simulink model "EMPlanner_cs"  (R2020a)
settings: Solver=ode5  StartTime=0.0  StopTime=30  FixedStep=1/1000  RelTol=1e-3
PreLoadFcn:
  | mbxruntime.callbacks.PreLoadFcn(bdroot);
PostLoadFcn:
  | mbxruntime.callbacks.PostLoadFcn(bdroot);
InitFcn:
  | mbxruntime.callbacks.InitFcn(bdroot);
StartFcn:
  | mbxruntime.callbacks.StartFcn(bdroot);
StopFcn:
  | mbxruntime.callbacks.StopFcn(bdroot);
model workspace (MAT data in the model file):
  mbox_table : object (value not decoded)
  model_closed = 0
  sim_status = 0
values from neighbouring files (symbols this model uses):
  aubr = [-8 -7.95 -7.9 -7.85 -7.8 -7.75 -7.7 -7.65 -7.6 -7.55 -7.5 -7.45 ... (261 elements, 1x261)]    [table_calibration.mat]
  tablebr = [-1.5 -1.5 -6.69193204056 -6.72439369683 -6.74529114616 -6.75462438856 -6.75239342402 -6.74076432593 -6.71187451024 -6.7106900587 -6.78609036519 -6.73359919607 ... (261261 elements, 1001x261)]    [table_calibration.mat]
  vubr = [0 0.05 0.1 0.15 0.2 0.25 0.3 0.35 0.4 0.45 0.5 0.55 ... (1001 elements, 1x1001)]    [table_calibration.mat]
undefined symbols (not defined in the file or in its folder): c_factor, cf, cr, DiscIntNeverNeededParam, global_path_x, global_path_y, KD_PID_distance, KD_PID_speed, KI_PID_distance, KI_PID_speed, KP_PID_distance, KP_PID_speed, la, lb, LQR_K1, LQR_K2, LQR_K3, LQR_K4, m, rack_displacement, right_wheel_ground, vx_break_point, warningInitialVelocity, x0
libraries: PreScanSimulinkLibrary x39, simulink x19, simulink_extras x11, Solver_SF x1
(part 1 of 11)
CloseFcn:
  | mbxruntime.callbacks.CloseFcn(bdroot);
settings Model: EnablePacing=on  PacingRate=1000  Creator=PRESCAN  LastModifiedBy=vincentwong
settings DataIOCC: LimitDataPoints=on  SaveFormat=Array  ReturnWorkspaceOutputs=off
settings OptimizationCC: ExpressionDepthLimit=2147483647  InitFltsAndDblsToZero=on  LifeSpan=inf
settings DebuggingCC: SaveWithParameterizedLinksMsg=none  UnderspecifiedInitializationDetection=Classic  MergeDetectMultiDrivingBlocksExec=none  SignalResolutionControl=TryResolveAllWithWarning  MultiTaskDSMMsg=warning  MultiTaskCondExecSysMsg=none  FcnCallInpInsideContextMsg=warning  StateNameClashWarn=warning  SFUnexpectedBacktrackingDiag=warning  SFNoUnconditionalDefaultTransitionDiag=warning  SFExecutionAtInitializationDiag=none  ArithmeticOperatorsInVariantConditions=warning
settings HardwareCC: ProdBitPerPointer=32  ProdBitPerSizeT=32  ProdBitPerPtrDiffT=32  ProdLargestAtomicFloat=None  ProdIntDivRoundTo=Undefined  ProdEndianess=Unspecified  ProdWordSize=32  ProdHWDeviceType=32-bit Generic
settings ModelReferenceCC: UpdateModelReferenceTargets=IfOutOfDate  PropagateSignalLabelsOutOfModel=off
settings SFSimCC: SimUseLocalCustomCode=off  SimParseCustomCode=off  CustomCodeUndefinedFunction=UseInterfaceOnly
settings SFSimCC: SimCustomHeaderCode=|
  | #include "prescan.h"
  | #include "prescan_platform.h"
settings RTWCC: RTWUseLocalCustomCode=off
settings CodeAppCC: StateflowObjectComments=on
settings GRTTargetCC: TargetFcnLib=ansi_tfl_tmw.mat  TargetLangStandard=C89/C90 (ANSI)  CombineOutputUpdateFcns=off  GRTInterface=on
settings ConfigComp: CovMetricSettings=dw  CovSaveCumulativeToWorkspaceVar=on  CovSaveSingleToWorkspaceVar=on  CovExternalEMLEnable=off

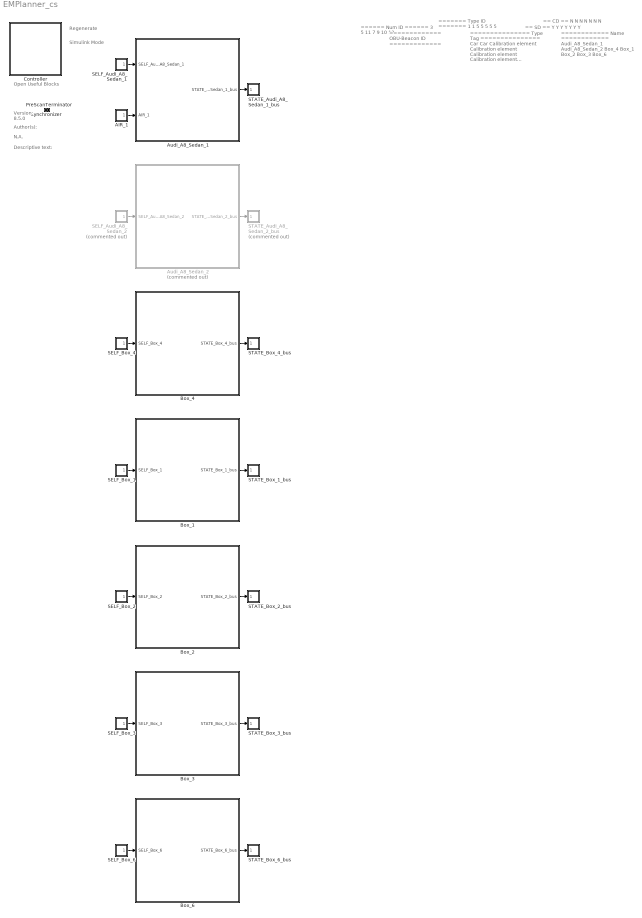
== system EMPlanner_cs ==
  note: Regenerate
  note: Simulink Mode
  note: Open Useful Blocks
  note: 8.5.0
  note: Version:
  note: Author(s):
  note: N.A.
  note: Descriptive text:
  note: ======
      | Num ID
      | ======
      | 3
      | 5
      | 11
      | 7
      | 9
      | 10
      | 13
  note: =============
      | OBU-Beacon ID
      | =============
  note: =======
      | Type ID
      | =======
      | 1
      | 1
      | 5
      | 5
      | 5
      | 5
      | 5
  note: ===============
      | Type Tag
      | ===============
      | Car
      | Car
      | Calibration element
      | Calibration element
      | Calibration element
      | Calibration element
      | Calibration element
  note: ==
      | SD
      | ==
      | Y
      | Y
      | Y
      | Y
      | Y
      | Y
      | Y
  note: ==
      | CD
      | ==
      | N
      | N
      | N
      | N
      | N
      | N
      | N
  note: ============
      | Name
      | ============
      | Audi_A8_Sedan_1
      | Audi_A8_Sedan_2
      | Box_4
      | Box_1
      | Box_2
      | Box_3
      | Box_6
  AIR_1 : Subsystem  Tag=sensor/AIR  Priority=3  LoadFcn=load('PrescanAIRSensorData.mat');load('PrescanAIRSensorMessage.mat')  mask(PreScan Source Block: Actor Independent Receiver (AIR)){}
      mask help:
      | The Actor Information Receiver sensor provides a fast, simple and generic detection solution which is not tied up to a specific technology. The AIR detects the intersection point of the bounding box with the straight line from the sensor axis system to the middle of the bounding box.
      |
      | For more information, please click Help.
      settings: OpenFcn=open_system([gcb '/Sensor'],'mask')
      mask Help: eval('openHelp(413)')
      mask Display: image(imread('AIR.png'))
  Audi_A8_Sedan_1 : Subsystem  Tag=WorldObjectSubSystem  InitFcn=UniqueId = '22';
      mask init:
      | modelPath = GenericModelHelper.getGenericModelFilePath('ModelDepo','Vehicles\Audi_A8\Audi_A8.pgmb','d771622804618130053427da08a6d484');imagePath = GenericModelHelper.getCompilationPicture(modelPath, 'Audi_A8_HighPoly.png');
      mask Display: image(imread(imagePath));color('white');text(0, 0, ' ID=3\n')
  Audi_A8_Sedan_2 : Subsystem  Tag=WorldObjectSubSystem  Commented=on  InitFcn=UniqueId = '97';
      mask init: same as EMPlanner_cs/Audi_A8_Sedan_1
      mask Display: image(imread(imagePath));color('white');text(0, 0, ' ID=5\n')
  Box_1 : Subsystem  Tag=WorldObjectSubSystem  InitFcn=UniqueId = '663';
      mask init:
      | imagePath=which('Box.jpg');
      mask Display: image(imread(imagePath));color('white');text(0, 0, ' ID=7\n')
  Box_2 : Subsystem  Tag=WorldObjectSubSystem  InitFcn=UniqueId = '666';
      mask init:
      | imagePath=which('Box.jpg');
      mask Display: image(imread(imagePath));color('white');text(0, 0, ' ID=9\n')
  Box_3 : Subsystem  Tag=WorldObjectSubSystem  InitFcn=UniqueId = '669';
      mask init:
      | imagePath=which('Box.jpg');
      mask Display: image(imread(imagePath));color('white');text(0, 0, ' ID=10\n')
  Box_4 : Subsystem  Tag=WorldObjectSubSystem  InitFcn=UniqueId = '412';
      mask init:
      | imagePath=which('Box.jpg');
      mask Display: image(imread(imagePath));color('white');text(0, 0, ' ID=11\n')
  Box_6 : Subsystem  Tag=WorldObjectSubSystem  InitFcn=UniqueId = '675';
      mask init:
      | imagePath=which('Box.jpg');
      mask Display: image(imread(imagePath));color('white');text(0, 0, ' ID=13\n')
  Controller : Subsystem  Description=372990EE13D66FA494953D7C7A6571B9D9BF5D2CCB90BB414698C9FA1010E28A  Priority=-1  LoadFcn=load PreScanControllerData  mask(PreScan Simulation Controller){prescanversion='8.5.0', ModelReferencing=off, TimeStep=50/1000, ControlMode=0, PreScanExecutionMode=on, ControllerCount=0, ControllerIndex=0, ControllerOptions=''}
      mask prompts: prescanversion "PreScan Version"; ModelReferencing "Use Model Referencing"; TimeStep "Upload Period [s]"; ControlMode "Control Mode"; PreScanExecutionMode "Execution Mode"; ControllerCount "Controller Count"; ControllerIndex "Controller Index"; ControllerOptions "Controller Options"
      mask help:
      | Please do not remove this block from the compilation sheet,
      | as it connects the model to the PreScan environment.
      mask init:
      | model = bdroot(gcb);
      | ExperimentFile = mbxruntime.findExperimentFile(model,true); %relative path
      | 
      | [d1, d2, d3, prescandata] = prescan_Settings();
      | ModelDepo = fullfile(prescandata,'ModelDepo'); 
      | 
      | RTmode = mbxruntime.getRTMode(model);
      | 
      | SimulationMode = get_param(bdroot,'SimulationMode');
      | if strcmp(SimulationMode, 'rapid-accelerator')
      |     SimulationMode = 'external';
      | end
      | TargetName = get_param(bdroot,'SystemTargetFile');
      settings: ModelCloseFcn=assignin('base',['model_closed_' bdroot],true);
      mask Help: eval('openHelp(812)')
      mask Display: image(imread('prescanlogo.ico'))
  PreScanTerminator : Subsystem  Tag=PreScanTerminator  Priority=999  LoadFcn=load PrescanTerminatorData  mask(PreScan Simulation Terminator){TimeStep=50/1000}
      mask prompts: TimeStep "Upload Period [s]"
      mask help:
      | Please do not remove this block from the compilation sheet as it
      | connects the model to the PreScan environment.
      mask Help: eval('openHelp(812)')
      mask Display: image(imread('prescanlogo.ico'))
  SELF_Audi_A8_Sedan_1 : Subsystem  Tag=sensor/SelfPort  Priority=3  LoadFcn=load('PreScanSelfSensorData.mat')  mask(PreScan Source Block: SELF){}
      mask help:
      | The SELF port shows (state) information of the actor itself. The outputs are position in the experiment's axis system and the GPS coordinates, and the object's absolute velocity and compass heading.
      |
      | For more information, please click Help.
      settings: OpenFcn=open_system([gcb '/Sensor'],'mask')
      mask Help: eval('openHelp(462)')
      mask Display: image(imread('GPS.png'))
  SELF_Audi_A8_Sedan_2 : Subsystem  Tag=sensor/SelfPort  Priority=3  Commented=on  LoadFcn=load('PreScanSelfSensorData.mat')  mask(PreScan Source Block: SELF){}
      mask help:
      | The SELF port shows (state) information of the actor itself. The outputs are position in the experiment's axis system and the GPS coordinates, and the object's absolute velocity and compass heading.
      |
      | For more information, please click Help.
      settings: OpenFcn=open_system([gcb '/Sensor'],'mask')
      mask Help: eval('openHelp(462)')
      mask Display: image(imread('GPS.png'))
  SELF_Box_1 : Subsystem  Tag=sensor/SelfPort  Priority=3  LoadFcn=load('PreScanSelfSensorData.mat')  mask(PreScan Source Block: SELF){}
      mask help:
      | The SELF port shows (state) information of the actor itself. The outputs are position in the experiment's axis system and the GPS coordinates, and the object's absolute velocity and compass heading.
      |
      | For more information, please click Help.
      settings: OpenFcn=open_system([gcb '/Sensor'],'mask')
      mask Help: eval('openHelp(462)')
      mask Display: image(imread('GPS.png'))
  SELF_Box_2 : Subsystem  Tag=sensor/SelfPort  Priority=3  LoadFcn=load('PreScanSelfSensorData.mat')  mask(PreScan Source Block: SELF){}
      mask help:
      | The SELF port shows (state) information of the actor itself. The outputs are position in the experiment's axis system and the GPS coordinates, and the object's absolute velocity and compass heading.
      |
      | For more information, please click Help.
      settings: OpenFcn=open_system([gcb '/Sensor'],'mask')
      mask Help: eval('openHelp(462)')
      mask Display: image(imread('GPS.png'))
  SELF_Box_3 : Subsystem  Tag=sensor/SelfPort  Priority=3  LoadFcn=load('PreScanSelfSensorData.mat')  mask(PreScan Source Block: SELF){}
      mask help:
      | The SELF port shows (state) information of the actor itself. The outputs are position in the experiment's axis system and the GPS coordinates, and the object's absolute velocity and compass heading.
      |
      | For more information, please click Help.
      settings: OpenFcn=open_system([gcb '/Sensor'],'mask')
      mask Help: eval('openHelp(462)')
      mask Display: image(imread('GPS.png'))
  SELF_Box_4 : Subsystem  Tag=sensor/SelfPort  Priority=3  LoadFcn=load('PreScanSelfSensorData.mat')  mask(PreScan Source Block: SELF){}
      mask help:
      | The SELF port shows (state) information of the actor itself. The outputs are position in the experiment's axis system and the GPS coordinates, and the object's absolute velocity and compass heading.
      |
      | For more information, please click Help.
      settings: OpenFcn=open_system([gcb '/Sensor'],'mask')
      mask Help: eval('openHelp(462)')
      mask Display: image(imread('GPS.png'))
  SELF_Box_6 : Subsystem  Tag=sensor/SelfPort  Priority=3  LoadFcn=load('PreScanSelfSensorData.mat')  mask(PreScan Source Block: SELF){}
      mask help:
      | The SELF port shows (state) information of the actor itself. The outputs are position in the experiment's axis system and the GPS coordinates, and the object's absolute velocity and compass heading.
      |
      | For more information, please click Help.
      settings: OpenFcn=open_system([gcb '/Sensor'],'mask')
      mask Help: eval('openHelp(462)')
      mask Display: image(imread('GPS.png'))
  STATE_Audi_A8_Sedan_1_bus : Subsystem  Tag=actuator/StatePort  Priority=0  LoadFcn=load('PreScanStateActuatorData.mat')  mask(PreScan Sink Block: State){}
      mask help:
      | The Actor State contains a vector signal of size (9x1), containing the following signals:
      |
      | -  Position    	(x,y,z)             	[m]
      | -  Velocity    	(vx,vy,vz)         	[m/s]
      | -  Angles       	(Roll, Pitch, Yaw)	[rad]
      |
      | The Actor state is defined in the global axis system.
      | The state is superponed on the Initial position defined in the GUI.
      |
      | For more information, please click Help.
      settings: OpenFcn=open_system([gcb '/Actuator'],'mask')
      mask Help: eval('openHelp(222)')
      mask Display: image(imread('State.png'))
  STATE_Audi_A8_Sedan_2_bus : Subsystem  Tag=actuator/StatePort  Priority=0  Commented=on  LoadFcn=load('PreScanStateActuatorData.mat')  mask(PreScan Sink Block: State){}
      mask help:
      | The Actor State contains a vector signal of size (9x1), containing the following signals:
      |
      | -  Position    	(x,y,z)             	[m]
      | -  Velocity    	(vx,vy,vz)         	[m/s]
      | -  Angles       	(Roll, Pitch, Yaw)	[rad]
      |
      | The Actor state is defined in the global axis system.
      | The state is superponed on the Initial position defined in the GUI.
      |
      | For more information, please click Help.
      settings: OpenFcn=open_system([gcb '/Actuator'],'mask')
      mask Help: eval('openHelp(222)')
      mask Display: image(imread('State.png'))
  STATE_Box_1_bus : Subsystem  Tag=actuator/StatePort  Priority=0  LoadFcn=load('PreScanStateActuatorData.mat')  mask(PreScan Sink Block: State){}
      mask help:
      | The Actor State contains a vector signal of size (9x1), containing the following signals:
      |
      | -  Position    	(x,y,z)             	[m]
      | -  Velocity    	(vx,vy,vz)         	[m/s]
      | -  Angles       	(Roll, Pitch, Yaw)	[rad]
      |
      | The Actor state is defined in the global axis system.
      | The state is superponed on the Initial position defined in the GUI.
      |
      | For more information, please click Help.
      settings: OpenFcn=open_system([gcb '/Actuator'],'mask')
      mask Help: eval('openHelp(222)')
      mask Display: image(imread('State.png'))
  STATE_Box_2_bus : Subsystem  Tag=actuator/StatePort  Priority=0  LoadFcn=load('PreScanStateActuatorData.mat')  mask(PreScan Sink Block: State){}
      mask help:
      | The Actor State contains a vector signal of size (9x1), containing the following signals:
      |
      | -  Position    	(x,y,z)             	[m]
      | -  Velocity    	(vx,vy,vz)         	[m/s]
      | -  Angles       	(Roll, Pitch, Yaw)	[rad]
      |
      | The Actor state is defined in the global axis system.
      | The state is superponed on the Initial position defined in the GUI.
      |
      | For more information, please click Help.
      settings: OpenFcn=open_system([gcb '/Actuator'],'mask')
      mask Help: eval('openHelp(222)')
      mask Display: image(imread('State.png'))
  STATE_Box_3_bus : Subsystem  Tag=actuator/StatePort  Priority=0  LoadFcn=load('PreScanStateActuatorData.mat')  mask(PreScan Sink Block: State){}
      mask help:
      | The Actor State contains a vector signal of size (9x1), containing the following signals:
      |
      | -  Position    	(x,y,z)             	[m]
      | -  Velocity    	(vx,vy,vz)         	[m/s]
      | -  Angles       	(Roll, Pitch, Yaw)	[rad]
      |
      | The Actor state is defined in the global axis system.
      | The state is superponed on the Initial position defined in the GUI.
      |
      | For more information, please click Help.
      settings: OpenFcn=open_system([gcb '/Actuator'],'mask')
      mask Help: eval('openHelp(222)')
      mask Display: image(imread('State.png'))
  STATE_Box_4_bus : Subsystem  Tag=actuator/StatePort  Priority=0  LoadFcn=load('PreScanStateActuatorData.mat')  mask(PreScan Sink Block: State){}
      mask help:
      | The Actor State contains a vector signal of size (9x1), containing the following signals:
      |
      | -  Position    	(x,y,z)             	[m]
      | -  Velocity    	(vx,vy,vz)         	[m/s]
      | -  Angles       	(Roll, Pitch, Yaw)	[rad]
      |
      | The Actor state is defined in the global axis system.
      | The state is superponed on the Initial position defined in the GUI.
      |
      | For more information, please click Help.
      settings: OpenFcn=open_system([gcb '/Actuator'],'mask')
      mask Help: eval('openHelp(222)')
      mask Display: image(imread('State.png'))
  STATE_Box_6_bus : Subsystem  Tag=actuator/StatePort  Priority=0  LoadFcn=load('PreScanStateActuatorData.mat')  mask(PreScan Sink Block: State){}
      mask help:
      | The Actor State contains a vector signal of size (9x1), containing the following signals:
      |
      | -  Position    	(x,y,z)             	[m]
      | -  Velocity    	(vx,vy,vz)         	[m/s]
      | -  Angles       	(Roll, Pitch, Yaw)	[rad]
      |
      | The Actor state is defined in the global axis system.
      | The state is superponed on the Initial position defined in the GUI.
      |
      | For more information, please click Help.
      settings: OpenFcn=open_system([gcb '/Actuator'],'mask')
      mask Help: eval('openHelp(222)')
      mask Display: image(imread('State.png'))
  Synchronizer : Subsystem  Tag=PreScanSynchronizer  Priority=1  LoadFcn=load PrescanSynchronizeData  mask(PreScan Simulation Core Block){TimeStep=50/1000}
      mask prompts: TimeStep "Timestep [s]"
      mask help:
      | Please do not remove this block from the PreScan compilation sheet,
      | as it contains essential configuration parameters for a PreScan simulation.
      settings: DeleteFcn=PreScanBlockDeleteFcn;
      mask Display: image(imread('prescanlogo.ico'))
  wires:
  Audi_A8_Sedan_1/1(STATE_Audi_A8_Sedan_1_bus) -> STATE_Audi_A8_Sedan_1_bus/1(STATE_Audi_A8_Sedan_1_bus)
  SELF_Audi_A8_Sedan_1/1(SELF_Audi_A8_Sedan_1) -> Audi_A8_Sedan_1/1(SELF_Audi_A8_Sedan_1)
  AIR_1/1(AIR_1) -> Audi_A8_Sedan_1/2(AIR_1)
  Audi_A8_Sedan_2/1(STATE_Audi_A8_Sedan_2_bus) -> STATE_Audi_A8_Sedan_2_bus/1(STATE_Audi_A8_Sedan_2_bus)
  SELF_Audi_A8_Sedan_2/1(SELF_Audi_A8_Sedan_2) -> Audi_A8_Sedan_2/1(SELF_Audi_A8_Sedan_2)
  Box_4/1(STATE_Box_4_bus) -> STATE_Box_4_bus/1(STATE_Box_4_bus)
  SELF_Box_4/1(SELF_Box_4) -> Box_4/1(SELF_Box_4)
  Box_1/1(STATE_Box_1_bus) -> STATE_Box_1_bus/1(STATE_Box_1_bus)
  SELF_Box_1/1(SELF_Box_1) -> Box_1/1(SELF_Box_1)
  Box_2/1(STATE_Box_2_bus) -> STATE_Box_2_bus/1(STATE_Box_2_bus)
  SELF_Box_2/1(SELF_Box_2) -> Box_2/1(SELF_Box_2)
  Box_3/1(STATE_Box_3_bus) -> STATE_Box_3_bus/1(STATE_Box_3_bus)
  SELF_Box_3/1(SELF_Box_3) -> Box_3/1(SELF_Box_3)
  Box_6/1(STATE_Box_6_bus) -> STATE_Box_6_bus/1(STATE_Box_6_bus)
  SELF_Box_6/1(SELF_Box_6) -> Box_6/1(SELF_Box_6)

== system EMPlanner_cs/AIR_1 ==
  Sensor : S-Function  FunctionName=sfun_AIRSensor  Parameters=detectableObjects, sensorID, timestep  SFunctionDeploymentMode=off  EnableBusSupport=off  mask(PreScan Source Block: Actor Independent Receiver (AIR)){detectableObjects=32, sensorID=315, timestep=50/1000}
      mask prompts: detectableObjects "Max detectable objects"; sensorID "Sensor ID"; timestep "MATLAB timestep:"
      mask help:
      | The Actor Information Receiver sensor provides a fast, simple and generic detection solution which is not tied up to a specific technology. The AIR detects the intersection point of the bounding box with the straight line from the sensor axis system to the middle of the bounding box.
      |
      | For more information, please click Help.
      mask Help: eval('openHelp(413)')
      mask Display: image(imread('AIR.png'))
  AIR_1 : Outport  Tag=outport/AIR  OutDataTypeStr=Bus: PRESCAN_AIRSENSORMESSAGE  PortDimensions=32  SampleTime=50/1000
  wires:
  Sensor/1 -> AIR_1/1

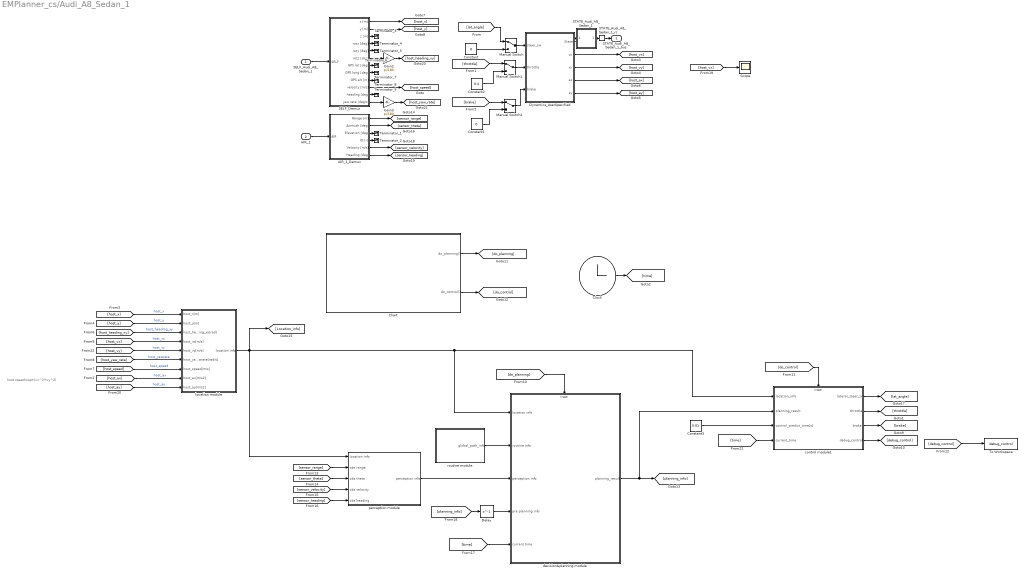
== system EMPlanner_cs/Audi_A8_Sedan_1 ==
  note: host speed=sqrt(vx^2+vy^2)
  SELF_Audi_A8_Sedan_1 : Inport  Tag=inport/SelfPort  OutDataTypeStr=Bus: PRESCAN_SELFSENSORDATA  PortDimensions=1  SampleTime=50/1000  BusOutputAsStruct=on
  AIR_1 : Inport  Tag=inport/AIR  Port=2  OutDataTypeStr=Bus: PRESCAN_AIRSENSORMESSAGE  PortDimensions=32  SampleTime=50/1000  BusOutputAsStruct=on
  AIR_1_Demux : Subsystem  Tag=demux/AIR  mask(PreScan Demux Block: AIR){DetectionType=CoG, detectableObjects=32}
      mask prompts: DetectionType "Detection Type"; detectableObjects "Max. detectable objects"
      mask help:
      | The Actor Information Receiver sensor provides a fast, simple and generic detection solution which is not tied up to a specific technology and can be used for scenarios in which a simple sensor is needed.
      |
      | For more information, please click Help.
      mask init:
      | switch DetectionType
      |     case 1
      |         DetectionTypeStr = 'Center';
      |     case 2
      |         DetectionTypeStr = 'BBox';
      |     case 3
      |         DetectionTypeStr = 'CoG';
      |     otherwise
      |         DetectionTypeStr = 'Unknown';
      | end
      settings: DeleteFcn=PreScanBlockDeleteFcn;
      mask Help: eval('openHelp(413)')
      mask TypeOptions DetectionType: Center | BBox | CoG
      mask Display:
      | disp(char('Det. type:         ',['{\it',DetectionTypeStr,'}']),'texmode','on')
      | port_label('output',1,'Range [m]')
      | port_label('output',2,'{\theta} [deg]','texmode','on')
      | port_label('output',3,'{\phi} [deg]','texmode','on')
      | port_label('output',4,'ID [-]','texmode','on')
      | port_label('output',5,'Velocity [m/s]','texmode','on')
      | port_label('output',6,'Heading [deg]','texmode','on')
  Chart : Stateflow chart  TreatAsAtomicUnit=on
  Clock : Clock
  Constant : Constant  Value=0
  Constant1 : Constant  Value=0
  Constant2 : Constant  Value=0.4
  Constant3 : Constant  Value=0.01
  Delay : Delay  DelayLength=1
  Dynamics_UserSpecified : Subsystem  Tag=UserSpecified_Subsys  Description=..\test_planning\Extensions\Simulink\CarSim_VehicleDynamics.mdl  mask(User specified subsystem){update=off, sourcefilename=..\test_planning\Extensions\Simulink\CarSim_VehicleDynamics.mdl}
      mask prompts: update "Update (default: not checked)"; sourcefilename "Source file name"
      mask help:
      | A User-specified model may be selected as Controller or Dynamics of the vehicle. PreScan will copy the contents of the User-specified model into the user-specified model block.
      |
      | If update checkbox is checked the current user-specified model block will be deleted and will be REPLACED by (new) user specified model blocks. So, the current user specified model elements will be lost.
      |
      | Warning: If a new user-specified model is selected in the GUI, the user-specified model will be replaced.
      settings: DeleteFcn=PreScanBlockDeleteFcn;
      mask Help: eval('openHelp(227)')
      mask Display: userSpecifiedDynamics_mask_display();
  Gain2 : Gain  Gain=pi/180
  Gain3 : Gain  Gain=pi/180
  Manual Switch : ManualSwitch
  Manual Switch1 : ManualSwitch
  Manual Switch2 : ManualSwitch
  SELF_Demux : Subsystem  Tag=demux/SelfPort  mask(PreScan Demux Block:){}
      mask help:
      | The SELF port shows (state) information of the actor itself. The outputs are position in the experiment's axis system and the GPS coordinates, and the object's absolute velocity and compass heading.
      |
      | For more information, please click Help.
      settings: DeleteFcn=PreScanBlockDeleteFcn;
      mask Help: eval('openHelp(462)')
      mask Display:
      | port_label('output',1,'x [m]')
      | port_label('output',2,'y [m]')
      | port_label('output',3,'z [m]','texmode','on')
      | port_label('output',4,'Rotx [deg]','texmode','on')
      | port_label('output',5,'Roty [deg]','texmode','on')
      | port_label('output',6,'Rotz [deg]','texmode','on')
      | port_label('output',7,'GPS lat [deg]','texmode','on')
      | port_label('output',8,'GPS long [deg]','texmode','on')
      | port_label('output',9,'GPS alt [m]','texmode','on')
      | port_label('output',10,'Velocity [m/s]')
      | port_label('output',11,'Heading [deg]')
      | port_label('output',12,'Yaw rate [deg/s]')
  STATE_Audi_A8_Sedan_1 : Subsystem  Tag=mux/StatePort  Priority=0  LoadFcn=load PrescanStateActuatorData  mask(PreScan Sink Block: State){x0=-1.0007, y0=2.7323, z0=0.55, Roll0=0, Pitch0=0, Yaw0=0, TimeStep=1/1000}
      mask prompts: x0 "Ini x-position VEHICLE wrt GLOBAL axis system [m]"; y0 "Ini y-position VEHICLE wrt GLOBAL axis system [m]"; z0 "Ini z-position VEHICLE wrt GLOBAL axis system [m]"; Roll0 "Ini roll-angle BODY wrt VEHICLE axis system [deg]"; Pitch0 "Ini pitch-angle BODY wrt VEHICLE axis system [deg]"; Yaw0 "Ini yaw-angle VEHICLE wrt GLOBAL axis system [deg]"; TimeStep "Auto-Assigned: Upload Period [s]"
      mask help:
      | The Actor State contains a vector signal of size (9x1), containing the following signals:
      |
      | -  Position                  (x,y,z)                                     [m]
      | -  Velocity                  (vx,vy,vz)                               [m/s]
      | -  Angles                    (Roll, Pitch, Yaw)                   [rad]
      |
      | The Actor state is defined in the global axis system.
      | The state is superponed on the Initial position defined in the GUI.
      |
      | For more information, please click Help.
      settings: DeleteFcn=PreScanBlockDeleteFcn;
      mask Help: eval('openHelp(222)')
      mask Display: image(imread('State.png'))
  STATE_Audi_A8_Sedan_1_rc : RateTransition  Tag=mux_rc/StatePort  OutPortSampleTimeOpt=Inherit
  Scope : Scope
  Terminator_{1..9} (9 alike) : Terminator
  To Workspace : ToWorkspace  VariableName=debug_control  SaveFormat=Timeseries  SampleTime=-1
  control module1 : Subsystem
  decision&planning module : Subsystem
  location module : Subsystem
  perception module : Subsystem
  routine module : Subsystem
  STATE_Audi_A8_Sedan_1_bus : Outport  Tag=outport/StatePort  OutDataTypeStr=Bus: PRESCAN_STATEACTUATORDATA  PortDimensions=1  SampleTime=50/1000
  wires:
  SELF_Demux/10(velocity [m/s]) -> [host_speed]
  SELF_Demux/1(x [m]) -> [host_x]
  SELF_Demux/6(rotz [deg]) -> Gain2/1
  SELF_Demux/12(yaw rate [deg/s]) -> Gain3/1
  Gain2/1 -> [host_heading_xy]
  Gain3/1 -> [host_yaw_rate]
  SELF_Demux/2(y [m]) -> [host_y]
  Dynamics_UserSpecified/2(vx) -> [host_vx]
  Dynamics_UserSpecified/3(vy) -> [host_vy]
  Dynamics_UserSpecified/5(ay) -> [host_ay]
  Dynamics_UserSpecified/4(ax) -> [host_ax]
  AIR_1_Demux/1(Range [m]) -> [sensor_range]
  AIR_1_Demux/2(Azimuth [deg]) -> [sensor_theta]
  AIR_1_Demux/5(Velocity [m/s]) -> [sensor_velocity]
  AIR_1_Demux/6(Heading [deg]) -> [sensor_heading]
  [lat_angle] -> Manual Switch/1
  Manual Switch/1 -> Dynamics_UserSpecified/1(steer_sw)
  Manual Switch1/1 -> Dynamics_UserSpecified/2(throttle)
  [throttle] -> Manual Switch1/1
  Manual Switch2/1 -> Dynamics_UserSpecified/3(brake)
  [brake] -> Manual Switch2/1
  Constant/1 -> Manual Switch/2
  Constant1/1 -> Manual Switch2/2
  Constant2/1 -> Manual Switch1/2
  [time] -> control module1/4(current_time)
  control module1/3(brake) -> [brake]
  [planning_info] -> Delay/1
  location module/1(location info) -> perception module/1(location info), decision&planning module/1(location info), control module1/1(location_info), [Location_info]
  Chart/2(do_control()) -> [do_control]
  [host_ay] -> location module/9(host_ay[m/s2])  "host_ay"
  [host_heading_xy] -> location module/3(host_heading_xy[rad])  "host_heading_xy"
  [sensor_range] -> perception module/2(obs range)
  [sensor_heading] -> perception module/5(obs heading)
  [host_ax] -> location module/8(host_ax[m/s2])  "host_ax"
  [do_control] -> control module1/Trigger
  [host_yaw_rate] -> location module/6(host_yawrate[rad/s])  "host_yawrate"
  Constant3/1 -> control module1/3(control_predict_time[s])
  [host_vx] -> location module/4(host_vx[m/s])  "host_vx"
  decision&planning module/1(planning_result) -> [planning_info], control module1/2(planning_result)
  control module1/1(lateral_steer_sw) -> [lat_angle]
  [do_planning] -> decision&planning module/Trigger
  [host_y] -> location module/2(host_y[m])  "host_y"
  control module1/4(debug_control) -> [debug_control]
  [time] -> decision&planning module/5(current time)
  routine module/1(global_path_info) -> decision&planning module/2(routine info)
  Clock/1 -> [time]
  control module1/2(throttle) -> [throttle]
  Chart/1(do_planning()) -> [do_planning]
  [sensor_theta] -> perception module/3(obs theta)
  [debug_control] -> To Workspace/1
  [host_x] -> location module/1(host_x[m])  "host_x"
  [host_vy] -> location module/5(host_vy[m/s])  "host_vy"
  [host_speed] -> location module/7(host_speed[m/s])  "host_speed"
  [sensor_velocity] -> perception module/4(obs velocity)
  perception module/1(perception info) -> decision&planning module/3(perception info)
  Delay/1 -> decision&planning module/4(pre planning info)
  [host_vx] -> Scope/1
  STATE_Audi_A8_Sedan_1_rc/1 -> STATE_Audi_A8_Sedan_1_bus/1
  STATE_Audi_A8_Sedan_1/1(StateBus) -> STATE_Audi_A8_Sedan_1_rc/1
  SELF_Audi_A8_Sedan_1/1 -> SELF_Demux/1(SELF)
  AIR_1/1 -> AIR_1_Demux/1(AIR)
  Dynamics_UserSpecified/1(State) -> STATE_Audi_A8_Sedan_1/1(State)
  AIR_1_Demux/3(Elevation [deg]) -> Terminator_1/1
  AIR_1_Demux/4(ID [-]) -> Terminator_2/1
  SELF_Demux/3(z [m]) -> Terminator_3/1
  SELF_Demux/4(rotx [deg]) -> Terminator_4/1
  SELF_Demux/5(roty [deg]) -> Terminator_5/1
  SELF_Demux/7(GPS lat [deg]) -> Terminator_6/1
  SELF_Demux/8(GPS long [deg]) -> Terminator_7/1
  SELF_Demux/9(GPS alt [m]) -> Terminator_8/1
  SELF_Demux/11(heading [deg]) -> Terminator_9/1

== system EMPlanner_cs/Audi_A8_Sedan_2 ==
  SELF_Audi_A8_Sedan_2 : Inport  Tag=inport/SelfPort  OutDataTypeStr=Bus: PRESCAN_SELFSENSORDATA  PortDimensions=1  SampleTime=50/1000  BusOutputAsStruct=on
  DesiredVelocity : Constant  Tag=DesiredVelocity  Value=15
  Dynamics_Simple : Subsystem  Tag=Simple_Vehicle_Dynamics  mask(PreScan Block: Simple Dynamics){Migrate=on, TimeStep=1/1000, ComputationMode=Continuous_Time}
      mask prompts: Migrate "Migrate. During migration this block will be replaced by a newer one."; TimeStep "Auto assigned: Time Step [s]"; ComputationMode "Computation mode:"
      mask help:
      | The Simple Dynamics Model is selected in the GUI to simulate vehicle dynamics behavior.
      |
      | The Simple Dynamics Model is completely open to the user. The parameters of this model can be set in the Simple Dynamics dialog in the GUI.
      |
      | For more information, please click Help.
      mask init:
      | p = SimpleDyn_pars;
      settings: DeleteFcn=PreScanBlockDeleteFcn;
      mask Help: eval('openHelp(220)')
      mask Display:
      | image(imread('SimpleDyn.png'))
      | port_label('input', 1, '{\delta}_S_t_ _e_e_r [deg]','texmode','on')
      | port_label('input', 2, 'Throttle [%]')
      | port_label('input', 3, 'Brake Pres [bar]')
      | port_label('input', 4, 'V_0 [ms-1]','texmode','on')
      | port_label('input', 5, 'Auto=[0]/Manual=[1]')
      | port_label('input', 6, 'Auto_GearShift')
      | port_label('input', 7, 'Manual_GearShift')
      | port_label('output', 1, 'State')
      | port_label('output', 2, 'Vx [ms-1]')
      | port_label('output', 3, 'Perf Params')
  FromDynamics2PathFollowerBusSelector : BusSelector  OutputSignals=vx_[ms-1],vy_[ms-1]
  Ground_1 : Ground
  Ground_2 : Ground
  Ground_3 : Ground
  InitialVelocity : Constant  Tag=InitialVelocity  Value=15
  PathFollower_Preview_1 : Subsystem  Tag=PathFollower_Preview  mask(PreScan Block: Path Follower with Preview){Migrate=on, LongCtrl_P=20, LongCtrl_I=0.3, LongCtrl_D=3.065, LongCtrl_AWU=1, LongCtrlDefault_P=20, LongCtrlDefault_I=0.3, LongCtrlDefault_D=3.065, LongCtrlDefault_AWU=1, FileName='Trajectory_1.mat', mass=1820, Jzz=3746, length_a=2.94 - 1.77, length_l=2.94, Angle_Max_SteeringWheel=500, PreviewTime=1, DelayTime=0.1, LowSpeedLimit=20, MaxSteeringRate=1200, CSSampleTime=1/1000, PFIntegrationFrequency=1000}
      mask prompts: Migrate "Migrate. During migration this block will be replaced by a newer one."; LongCtrl_P "Longitudinal Controller P"; LongCtrl_I "Longitudinal Controller I"; LongCtrl_D "Longitudinal Controller D"; LongCtrl_AWU "Longitudinal Controller AWU"; FileName "Trajectory Name"; mass "Mass vehicle total [kg]"; Jzz "Inertia vehicle around yaw axis [kg m2]"; length_a "Distance between COG and front axle [m]"; length_l "Length of wheelbase [m]"; Angle_Max_SteeringWheel "Maximum steering wheel angle [deg]"; PreviewTime "Preview time [s]"; DelayTime "Delay time [s]"; LowSpeedLimit "Low-speed limit [km/h]"; MaxSteeringRate "Maximum steering wheel angle rate [deg/s]"; CSSampleTime "Compilation Sheet sample time [s]"; PFIntegrationFrequency "Lateral controller frequency [Hz]"
      mask help:
      | The Path Follower Model is selected in the GUI to simulate driver behavior.
      |
      | For more information, please click Help.
      mask init:
      | load(['trajectories/',eval(FileName)])
      | traject=trajectory';
      | 
      | Traj_x=traject(:,2);
      | Traj_y=traject(:,3);
      | Traj_t=traject(2,1);
      | Traj_v=sqrt(traject(:,8).^2+traject(:,9).^2+traject(:,10).^2);
      | 
      | RefreshCounter = max(floor((1/CSSampleTime) / (PFIntegrationFrequency)), 1); %Compilation sheet frequency/path follower frequency
      | 
      | blockPath = gcb;
      | 
      | clear traject;
      mask Help: eval('openHelp(233)')
      mask DialogControl Container12 Prompt: Controller Parameters
      mask DialogControl Control2 Prompt: Reset PID parameters
      mask DialogControl Control2 Callback:
      | LongCtrlDefault_P = get_param(gcb,'LongCtrlDefault_P');
      | set_param(gcb,'LongCtrl_P',LongCtrlDefault_P);
      | 
      | LongCtrlDefault_I = get_param(gcb,'LongCtrlDefault_I');
      | set_param(gcb,'LongCtrl_I',LongCtrlDefault_I);
      | 
      | LongCtrlDefault_D = get_param(gcb,'LongCtrlDefault_D');
      | set_param(gcb,'LongCtrl_D',LongCtrlDefault_D);
      | 
      | LongCtrlDefault_AWU = get_param(gcb,'LongCtrlDefault_AWU');
      | set_param(gcb,'LongCtrl_AWU',LongCtrlDefault_AWU);
      mask DialogControl Container10 Prompt: System Parameters
  SELF_Demux : Subsystem  Tag=demux/SelfPort  mask(PreScan Demux Block:){}
      mask help:
      | The SELF port shows (state) information of the actor itself. The outputs are position in the experiment's axis system and the GPS coordinates, and the object's absolute velocity and compass heading.
      |
      | For more information, please click Help.
      settings: DeleteFcn=PreScanBlockDeleteFcn;
      mask Help: eval('openHelp(462)')
      mask Display:
      | port_label('output',1,'x [m]')
      | port_label('output',2,'y [m]')
      | port_label('output',3,'z [m]','texmode','on')
      | port_label('output',4,'Rotx [deg]','texmode','on')
      | port_label('output',5,'Roty [deg]','texmode','on')
      | port_label('output',6,'Rotz [deg]','texmode','on')
      | port_label('output',7,'GPS lat [deg]','texmode','on')
      | port_label('output',8,'GPS long [deg]','texmode','on')
      | port_label('output',9,'GPS alt [m]','texmode','on')
      | port_label('output',10,'Velocity [m/s]')
      | port_label('output',11,'Heading [deg]')
      | port_label('output',12,'Yaw rate [deg/s]')
  STATE_Audi_A8_Sedan_2 : Subsystem  Tag=mux/StatePort  Priority=0  LoadFcn=load PrescanStateActuatorData  mask(PreScan Sink Block: State){x0=-30.6672, y0=0.44913, z0=0.55, Roll0=0, Pitch0=0, Yaw0=0, TimeStep=1/1000}
      mask prompts: x0 "Ini x-position VEHICLE wrt GLOBAL axis system [m]"; y0 "Ini y-position VEHICLE wrt GLOBAL axis system [m]"; z0 "Ini z-position VEHICLE wrt GLOBAL axis system [m]"; Roll0 "Ini roll-angle BODY wrt VEHICLE axis system [deg]"; Pitch0 "Ini pitch-angle BODY wrt VEHICLE axis system [deg]"; Yaw0 "Ini yaw-angle VEHICLE wrt GLOBAL axis system [deg]"; TimeStep "Auto-Assigned: Upload Period [s]"
      mask help:
      | The Actor State contains a vector signal of size (9x1), containing the following signals:
      |
      | -  Position                  (x,y,z)                                     [m]
      | -  Velocity                  (vx,vy,vz)                               [m/s]
      | -  Angles                    (Roll, Pitch, Yaw)                   [rad]
      |
      | The Actor state is defined in the global axis system.
      | The state is superponed on the Initial position defined in the GUI.
      |
      | For more information, please click Help.
      settings: DeleteFcn=PreScanBlockDeleteFcn;
      mask Help: eval('openHelp(222)')
      mask Display: image(imread('State.png'))
  STATE_Audi_A8_Sedan_2_rc : RateTransition  Tag=mux_rc/StatePort  OutPortSampleTimeOpt=Inherit
  State2PathFollowerCnv : Subsystem  Tag=State2PFConnection/cnv
  Terminator_{1..14} (14 alike) : Terminator
  To Workspace : ToWorkspace  VariableName=global_path_x_original  SaveFormat=Timeseries  SampleTime=0.1
  To Workspace1 : ToWorkspace  VariableName=global_path_y_original  SaveFormat=Timeseries  SampleTime=0.1
  Trajectories : Subsystem  Tag=Trajectories  mask(PreScan Source Block: Trajectories){}
      mask help:
      | The Trajectory block contains the trajectories defined in the PreScan Experiment Editor. The output of the trajectory block is the (vehicle) State.
      |
      | For more information, please click Help.
      settings: DeleteFcn=PreScanBlockDeleteFcn;
      mask Help: eval('openHelp(312)')
      mask Display: image(imread('Trajectory.png'));
  pos : Constant  Tag=pos  Value=[-30.6672 0.44913 0]
  steering_ratio : Constant  Tag=steering_ratio  Value=20
  susp_front : Constant  Tag=susp_front  Value=72653
  susp_rear : Constant  Tag=susp_rear  Value=121449
  STATE_Audi_A8_Sedan_2_bus : Outport  Tag=outport/StatePort  OutDataTypeStr=Bus: PRESCAN_STATEACTUATORDATA  PortDimensions=1  SampleTime=50/1000
  wires:
  SELF_Demux/1(x [m]) -> To Workspace/1
  SELF_Demux/2(y [m]) -> To Workspace1/1
  STATE_Audi_A8_Sedan_2_rc/1 -> STATE_Audi_A8_Sedan_2_bus/1
  STATE_Audi_A8_Sedan_2/1(StateBus) -> STATE_Audi_A8_Sedan_2_rc/1, [State]
  SELF_Audi_A8_Sedan_2/1 -> SELF_Demux/1(SELF)
  pos/1 -> PathFollower_Preview_1/1(TrajOffset x,y,Y [m,m,deg])
  susp_front/1 -> PathFollower_Preview_1/10(CorneringStiffness_Tyres_Front [N/rad])
  susp_rear/1 -> PathFollower_Preview_1/11(CorneringStiffness_Tyres_Rear [N/rad])
  steering_ratio/1 -> PathFollower_Preview_1/12(steering_ratio[-])
  InitialVelocity/1 -> PathFollower_Preview_1/4(Initial Velocity [m/s])
  DesiredVelocity/1 -> PathFollower_Preview_1/5(Desired Velocity [m/s])
  [State] -> State2PathFollowerCnv/1(State BUS)
  State2PathFollowerCnv/1(Yaw rate [deg/s]) -> PathFollower_Preview_1/9(Yaw rate [deg/s])
  State2PathFollowerCnv/2(velocity [m/s]) -> PathFollower_Preview_1/6(velocity [m/s])
  State2PathFollowerCnv/3(position x,y,Y [m,m,deg]) -> PathFollower_Preview_1/3(position x,y,Y [m,m,deg])
  PathFollower_Preview_1/1(delta_steerwheel [deg]) -> Dynamics_Simple/1(DeltaSteer_[deg])
  PathFollower_Preview_1/2(throttle [%]) -> Dynamics_Simple/2(Throttle)
  PathFollower_Preview_1/3(brake pressure [bar]) -> Dynamics_Simple/3(Brake)
  PathFollower_Preview_1/4(v0 [m/s]) -> Dynamics_Simple/4(Initial_Vx_[ms-1])
  PathFollower_Preview_1/5(Auto_GearShift) -> Dynamics_Simple/6(Auto_GearShift)
  Dynamics_Simple/3(Perf_Params) -> [Dynamics2PathFollower]
  FromDynamics2PathFollowerBusSelector/1 -> PathFollower_Preview_1/7(vx [m/s])  "<vx_[ms-1]>"
  FromDynamics2PathFollowerBusSelector/2 -> PathFollower_Preview_1/8(vy [m/s])  "<vy_[ms-1]>"
  [Dynamics2PathFollower] -> FromDynamics2PathFollowerBusSelector/1
  Dynamics_Simple/1(State) -> STATE_Audi_A8_Sedan_2/1(State)
  Ground_1/1 -> Dynamics_Simple/5(AutoManual_OnOff)
  Ground_2/1 -> Dynamics_Simple/7(Manual_GearShift)
  Dynamics_Simple/2(Vx [m s-1]) -> Terminator_1/1
  Ground_3/1 -> PathFollower_Preview_1/2(ActorOffset_Left(+) / Right(-) [m])
  PathFollower_Preview_1/6(Actor/Traj_distance [m]) -> Terminator_2/1
  PathFollower_Preview_1/7(Actor/Traj_angle [deg]) -> Terminator_3/1
  SELF_Demux/3(z [m]) -> Terminator_4/1
  SELF_Demux/4(rotx [deg]) -> Terminator_5/1
  SELF_Demux/5(roty [deg]) -> Terminator_6/1
  SELF_Demux/6(rotz [deg]) -> Terminator_7/1
  SELF_Demux/7(GPS lat [deg]) -> Terminator_8/1
  SELF_Demux/8(GPS long [deg]) -> Terminator_9/1
  SELF_Demux/9(GPS alt [m]) -> Terminator_10/1
  SELF_Demux/10(velocity [m/s]) -> Terminator_11/1
  SELF_Demux/11(heading [deg]) -> Terminator_12/1
  SELF_Demux/12(yaw rate [deg/s]) -> Terminator_13/1
  Trajectories/1(State) -> Terminator_14/1

== system EMPlanner_cs/Box_1 ==
  SELF_Box_1 : Inport  Tag=inport/SelfPort  OutDataTypeStr=Bus: PRESCAN_SELFSENSORDATA  PortDimensions=1  SampleTime=50/1000  BusOutputAsStruct=on
  SELF_Demux : Subsystem  Tag=demux/SelfPort  mask(PreScan Demux Block:){}
      mask help:
      | The SELF port shows (state) information of the actor itself. The outputs are position in the experiment's axis system and the GPS coordinates, and the object's absolute velocity and compass heading.
      |
      | For more information, please click Help.
      settings: DeleteFcn=PreScanBlockDeleteFcn;
      mask Help: eval('openHelp(462)')
      mask Display:
      | port_label('output',1,'x [m]')
      | port_label('output',2,'y [m]')
      | port_label('output',3,'z [m]','texmode','on')
      | port_label('output',4,'Rotx [deg]','texmode','on')
      | port_label('output',5,'Roty [deg]','texmode','on')
      | port_label('output',6,'Rotz [deg]','texmode','on')
      | port_label('output',7,'GPS lat [deg]','texmode','on')
      | port_label('output',8,'GPS long [deg]','texmode','on')
      | port_label('output',9,'GPS alt [m]','texmode','on')
      | port_label('output',10,'Velocity [m/s]')
      | port_label('output',11,'Heading [deg]')
      | port_label('output',12,'Yaw rate [deg/s]')
  STATE_Box_1 : Subsystem  Tag=mux/StatePort  Priority=0  LoadFcn=load PrescanStateActuatorData  mask(PreScan Sink Block: State){x0=143.5395, y0=33.5841, z0=0, Roll0=0, Pitch0=0, Yaw0=270, TimeStep=50/1000}
      mask prompts: x0 "Ini x-position VEHICLE wrt GLOBAL axis system [m]"; y0 "Ini y-position VEHICLE wrt GLOBAL axis system [m]"; z0 "Ini z-position VEHICLE wrt GLOBAL axis system [m]"; Roll0 "Ini roll-angle BODY wrt VEHICLE axis system [deg]"; Pitch0 "Ini pitch-angle BODY wrt VEHICLE axis system [deg]"; Yaw0 "Ini yaw-angle VEHICLE wrt GLOBAL axis system [deg]"; TimeStep "Auto-Assigned: Upload Period [s]"
      mask help:
      | The Actor State contains a vector signal of size (9x1), containing the following signals:
      |
      | -  Position                  (x,y,z)                                     [m]
      | -  Velocity                  (vx,vy,vz)                               [m/s]
      | -  Angles                    (Roll, Pitch, Yaw)                   [rad]
      |
      | The Actor state is defined in the global axis system.
      | The state is superponed on the Initial position defined in the GUI.
      |
      | For more information, please click Help.
      settings: DeleteFcn=PreScanBlockDeleteFcn;
      mask Help: eval('openHelp(222)')
      mask Display: image(imread('State.png'))
  STATE_Box_1_rc : RateTransition  Tag=mux_rc/StatePort  OutPortSampleTimeOpt=Inherit
  Terminator_{1..12} (12 alike) : Terminator
  Trajectories : Subsystem  Tag=Trajectories  mask(PreScan Source Block: Trajectories){}
      mask help:
      | The Trajectory block contains the trajectories defined in the PreScan Experiment Editor. The output of the trajectory block is the (vehicle) State.
      |
      | For more information, please click Help.
      settings: DeleteFcn=PreScanBlockDeleteFcn;
      mask Help: eval('openHelp(312)')
      mask Display: image(imread('Trajectory.png'));
  STATE_Box_1_bus : Outport  Tag=outport/StatePort  OutDataTypeStr=Bus: PRESCAN_STATEACTUATORDATA  PortDimensions=1  SampleTime=50/1000
  wires:
  STATE_Box_1_rc/1 -> STATE_Box_1_bus/1
  STATE_Box_1/1(StateBus) -> STATE_Box_1_rc/1
  SELF_Box_1/1 -> SELF_Demux/1(SELF)
  Trajectories/1(State) -> STATE_Box_1/1(State)
  SELF_Demux/1(x [m]) -> Terminator_1/1
  SELF_Demux/2(y [m]) -> Terminator_2/1
  SELF_Demux/3(z [m]) -> Terminator_3/1
  SELF_Demux/4(rotx [deg]) -> Terminator_4/1
  SELF_Demux/5(roty [deg]) -> Terminator_5/1
  SELF_Demux/6(rotz [deg]) -> Terminator_6/1
  SELF_Demux/7(GPS lat [deg]) -> Terminator_7/1
  SELF_Demux/8(GPS long [deg]) -> Terminator_8/1
  SELF_Demux/9(GPS alt [m]) -> Terminator_9/1
  SELF_Demux/10(velocity [m/s]) -> Terminator_10/1
  SELF_Demux/11(heading [deg]) -> Terminator_11/1
  SELF_Demux/12(yaw rate [deg/s]) -> Terminator_12/1

== system EMPlanner_cs/Box_2 ==
  SELF_Box_2 : Inport  Tag=inport/SelfPort  OutDataTypeStr=Bus: PRESCAN_SELFSENSORDATA  PortDimensions=1  SampleTime=50/1000  BusOutputAsStruct=on
  SELF_Demux : Subsystem  Tag=demux/SelfPort  mask(PreScan Demux Block:){}
      mask help:
      | The SELF port shows (state) information of the actor itself. The outputs are position in the experiment's axis system and the GPS coordinates, and the object's absolute velocity and compass heading.
      |
      | For more information, please click Help.
      settings: DeleteFcn=PreScanBlockDeleteFcn;
      mask Help: eval('openHelp(462)')
      mask Display:
      | port_label('output',1,'x [m]')
      | port_label('output',2,'y [m]')
      | port_label('output',3,'z [m]','texmode','on')
      | port_label('output',4,'Rotx [deg]','texmode','on')
      | port_label('output',5,'Roty [deg]','texmode','on')
      | port_label('output',6,'Rotz [deg]','texmode','on')
      | port_label('output',7,'GPS lat [deg]','texmode','on')
      | port_label('output',8,'GPS long [deg]','texmode','on')
      | port_label('output',9,'GPS alt [m]','texmode','on')
      | port_label('output',10,'Velocity [m/s]')
      | port_label('output',11,'Heading [deg]')
      | port_label('output',12,'Yaw rate [deg/s]')
  STATE_Box_2 : Subsystem  Tag=mux/StatePort  Priority=0  LoadFcn=load PrescanStateActuatorData  mask(PreScan Sink Block: State){x0=198.5038, y0=32.2133, z0=0, Roll0=0, Pitch0=0, Yaw0=270, TimeStep=50/1000}
      mask prompts: x0 "Ini x-position VEHICLE wrt GLOBAL axis system [m]"; y0 "Ini y-position VEHICLE wrt GLOBAL axis system [m]"; z0 "Ini z-position VEHICLE wrt GLOBAL axis system [m]"; Roll0 "Ini roll-angle BODY wrt VEHICLE axis system [deg]"; Pitch0 "Ini pitch-angle BODY wrt VEHICLE axis system [deg]"; Yaw0 "Ini yaw-angle VEHICLE wrt GLOBAL axis system [deg]"; TimeStep "Auto-Assigned: Upload Period [s]"
      mask help:
      | The Actor State contains a vector signal of size (9x1), containing the following signals:
      |
      | -  Position                  (x,y,z)                                     [m]
      | -  Velocity                  (vx,vy,vz)                               [m/s]
      | -  Angles                    (Roll, Pitch, Yaw)                   [rad]
      |
      | The Actor state is defined in the global axis system.
      | The state is superponed on the Initial position defined in the GUI.
      |
      | For more information, please click Help.
      settings: DeleteFcn=PreScanBlockDeleteFcn;
      mask Help: eval('openHelp(222)')
      mask Display: image(imread('State.png'))
  STATE_Box_2_rc : RateTransition  Tag=mux_rc/StatePort  OutPortSampleTimeOpt=Inherit
  Terminator_{1..12} (12 alike) : Terminator
  Trajectories : Subsystem  Tag=Trajectories  mask(PreScan Source Block: Trajectories){}
      mask help:
      | The Trajectory block contains the trajectories defined in the PreScan Experiment Editor. The output of the trajectory block is the (vehicle) State.
      |
      | For more information, please click Help.
      settings: DeleteFcn=PreScanBlockDeleteFcn;
      mask Help: eval('openHelp(312)')
      mask Display: image(imread('Trajectory.png'));
  STATE_Box_2_bus : Outport  Tag=outport/StatePort  OutDataTypeStr=Bus: PRESCAN_STATEACTUATORDATA  PortDimensions=1  SampleTime=50/1000
  wires:
  STATE_Box_2_rc/1 -> STATE_Box_2_bus/1
  STATE_Box_2/1(StateBus) -> STATE_Box_2_rc/1
  SELF_Box_2/1 -> SELF_Demux/1(SELF)
  Trajectories/1(State) -> STATE_Box_2/1(State)
  SELF_Demux/1(x [m]) -> Terminator_1/1
  SELF_Demux/2(y [m]) -> Terminator_2/1
  SELF_Demux/3(z [m]) -> Terminator_3/1
  SELF_Demux/4(rotx [deg]) -> Terminator_4/1
  SELF_Demux/5(roty [deg]) -> Terminator_5/1
  SELF_Demux/6(rotz [deg]) -> Terminator_6/1
  SELF_Demux/7(GPS lat [deg]) -> Terminator_7/1
  SELF_Demux/8(GPS long [deg]) -> Terminator_8/1
  SELF_Demux/9(GPS alt [m]) -> Terminator_9/1
  SELF_Demux/10(velocity [m/s]) -> Terminator_10/1
  SELF_Demux/11(heading [deg]) -> Terminator_11/1
  SELF_Demux/12(yaw rate [deg/s]) -> Terminator_12/1
